simulink model "main"  (R2016b)
settings: Solver=VariableStepAuto  StartTime=0.0  StopTime=40  FixedStep=Par.Step_size  RelTol=1e-3
values from neighbouring files (symbols this model uses):
  eta_0 = [0 0 0]    [K_psi_test.m]
  nu_0 = [0 0 0]    [K_psi_test.m]
undefined symbols (not defined in the file or in its folder): now, Par
libraries: simulink x4
settings Model: Creator=Ørjan  LastModifiedBy=Ørjan
settings DataIOCC: SaveState=on  ReturnWorkspaceOutputs=on  ReturnWorkspaceOutputsName=spidata
settings RTWCC: RTWCompilerOptimization=on
settings CodeAppCC: MaxIdLength=95

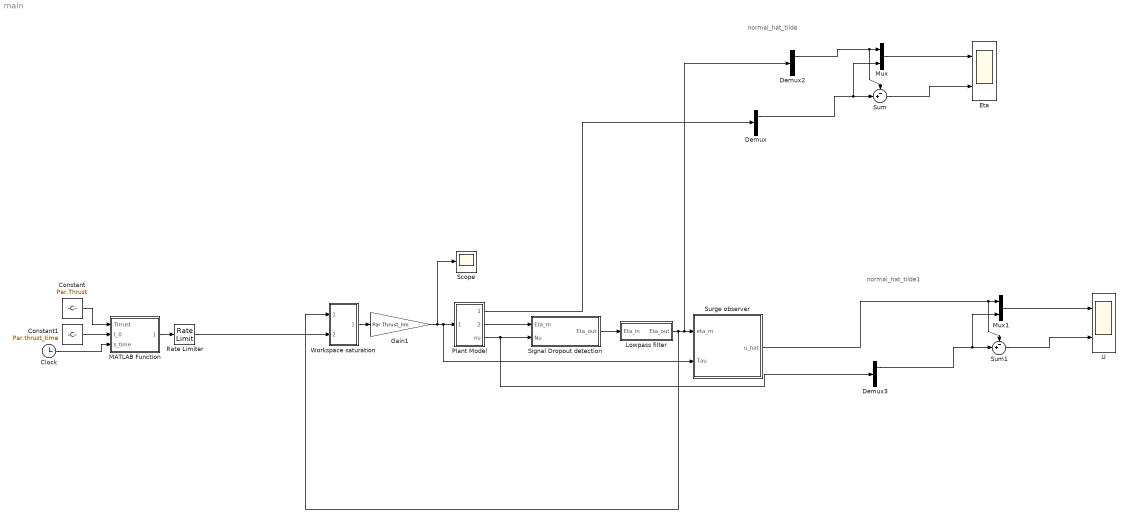
== system main ==
  note: normal_hat_tilde1
  note: normal_hat_tilde
  Clock : Clock
  Constant : Constant  Value=Par.Thrust  VectorParams1D=off
  Constant1 : Constant  Value=Par.thrust_time
  Demux : Demux  Outputs=3
  Demux2 : Demux  Outputs=3
  Demux3 : Demux  Outputs=3
  Eta : Scope  NumInputPorts=2
  Gain1 : Gain  Gain=Par.Thrust_lim
  Lowpass filter : Subsystem
  MATLAB Function : MATLAB Function  TreatAsAtomicUnit=on
  Mux : Mux  Inputs=2
  Mux1 : Mux  Inputs=2
  Plant Model : Subsystem
  Rate Limiter : RateLimiter  RisingSlewLimit=5  FallingSlewLimit=-5  SampleTimeMode=inherited
  Scope : Scope
  Signal Dropout detection : Subsystem
  Sum : Sum  Inputs=-+|
  Sum1 : Sum  Inputs=-+|
  Surge observer : Subsystem
  U : Scope  NumInputPorts=2
  Workspace saturation : Subsystem
  wires:
  Constant/1 -> MATLAB Function/1(Thrust)
  Clock/1 -> MATLAB Function/3(s_time)
  MATLAB Function/1(tau_norm) -> Rate Limiter/1
  Rate Limiter/1 -> Workspace saturation/2(Tau_in)
  Workspace saturation/1(Tau_out) -> Gain1/1
  Plant Model/2(eta_m) -> Signal Dropout detection/1(Eta_m)
  Signal Dropout detection/1(Eta_out) -> Lowpass filter/1(Eta_in)
  Gain1/1 -> Scope/1, Surge observer/2(Tau), Plant Model/1(tau)
  Lowpass filter/1(Eta_out) -> Workspace saturation/1(Eta_in), Demux2/1, Surge observer/1(eta_m)
  Plant Model/1(eta) -> Demux/1
  Demux/1 -> Mux/2, Sum/2
  Sum/1 -> Eta/2
  Demux2/1 -> Sum/1, Mux/1
  Mux/1 -> Eta/1
  Plant Model/3(nu) -> Demux3/1, Signal Dropout detection/2(Nu)
  Demux3/1 -> Mux1/2, Sum1/2
  Sum1/1 -> U/2
  Surge observer/1(u_hat) -> Sum1/1, Mux1/1
  Mux1/1 -> U/1
  Constant1/1 -> MATLAB Function/2(t_0)

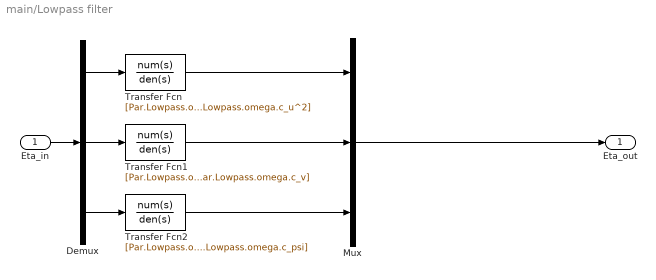
== system main/Lowpass filter ==
  Eta_in : Inport
  Demux : Demux  Outputs=3
  Mux : Mux  Inputs=3
  Transfer Fcn : TransferFcn  Numerator=[Par.Lowpass.omega.c_u^2]  Denominator=[1 Par.Lowpass.omega.c_u Par.Lowpass.omega.c_u^2]
  Transfer Fcn1 : TransferFcn  Numerator=[Par.Lowpass.omega.c_v]  Denominator=[1 Par.Lowpass.omega.c_v]
  Transfer Fcn2 : TransferFcn  Numerator=[Par.Lowpass.omega.c_psi]  Denominator=[1 Par.Lowpass.omega.c_psi]
  Eta_out : Outport
  wires:
  Eta_in/1 -> Demux/1
  Demux/1 -> Transfer Fcn/1
  Demux/2 -> Transfer Fcn1/1
  Demux/3 -> Transfer Fcn2/1
  Transfer Fcn2/1 -> Mux/3
  Transfer Fcn1/1 -> Mux/2
  Transfer Fcn/1 -> Mux/1
  Mux/1 -> Eta_out/1

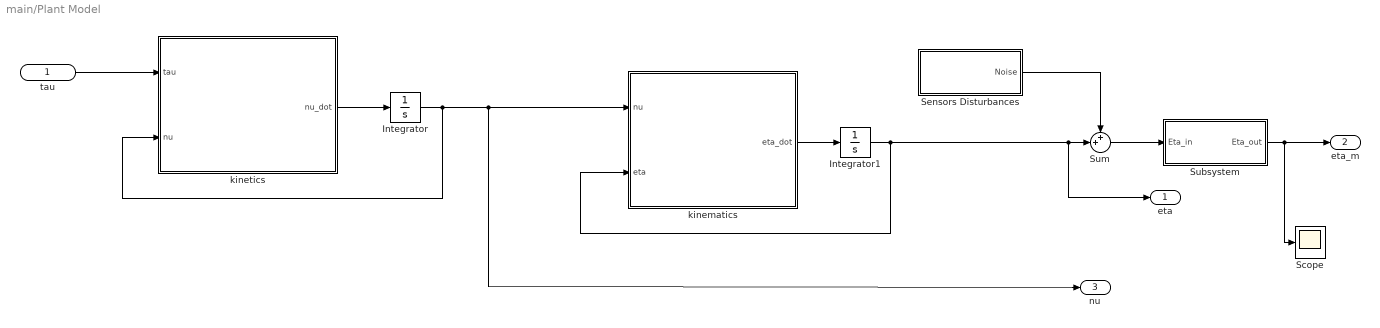
== system main/Plant Model ==
  tau : Inport
  Integrator : Integrator  InitialCondition=nu_0
  Integrator1 : Integrator  InitialCondition=eta_0
  Scope : Scope
  Sensors Disturbances : Subsystem
  Subsystem : Subsystem
  Sum : Sum  Inputs=++|
  kinematics : MATLAB Function  TreatAsAtomicUnit=on
  kinetics : MATLAB Function  TreatAsAtomicUnit=on
  eta : Outport
  eta_m : Outport  Port=2
  nu : Outport  Port=3
  wires:
  tau/1 -> kinetics/1(tau)
  kinetics/1(nu_dot) -> Integrator/1
  kinematics/1(eta_dot) -> Integrator1/1
  Integrator/1 -> kinetics/2(nu), nu/1, kinematics/1(nu)
  Integrator1/1 -> eta/1, Sum/2, kinematics/2(eta)
  Sensors Disturbances/1(Noise) -> Sum/1
  Subsystem/1(Eta_out) -> Scope/1, eta_m/1
  Sum/1 -> Subsystem/1(Eta_in)

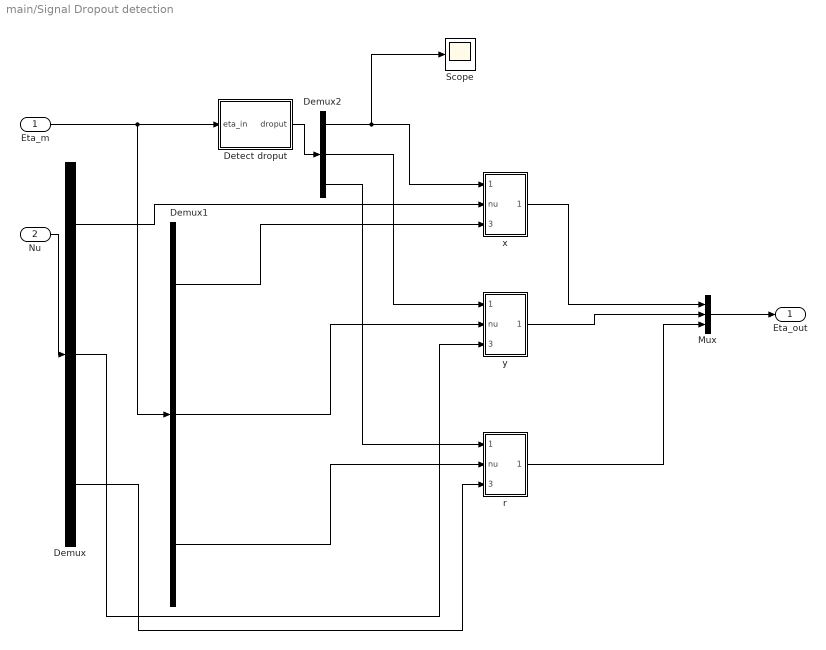
== system main/Signal Dropout detection ==
  Eta_m : Inport
  Nu : Inport  Port=2
  Demux : Demux  Outputs=3
  Demux1 : Demux  Outputs=3
  Demux2 : Demux  Outputs=3
  Detect droput : MATLAB Function  TreatAsAtomicUnit=on
  Mux : Mux  Inputs=3
  Scope : Scope
  r : Subsystem
  x : Subsystem
  y : Subsystem
  Eta_out : Outport
  wires:
  Nu/1 -> Demux/1
  Eta_m/1 -> Detect droput/1(eta_in), Demux1/1
  Detect droput/1(droput) -> Demux2/1
  y/1(new_eta) -> Mux/2
  r/1(new_eta) -> Mux/3
  Mux/1 -> Eta_out/1
  Demux2/1 -> Scope/1, x/1(detect droput)
  Demux/1 -> x/2(nu)
  Demux1/1 -> x/3(eta)
  x/1(new_eta) -> Mux/1
  Demux1/2 -> y/2(nu)
  Demux2/2 -> y/1(detect droput)
  Demux2/3 -> r/1(detect droput)
  Demux1/3 -> r/2(nu)
  Demux/2 -> y/3(eta)
  Demux/3 -> r/3(eta)

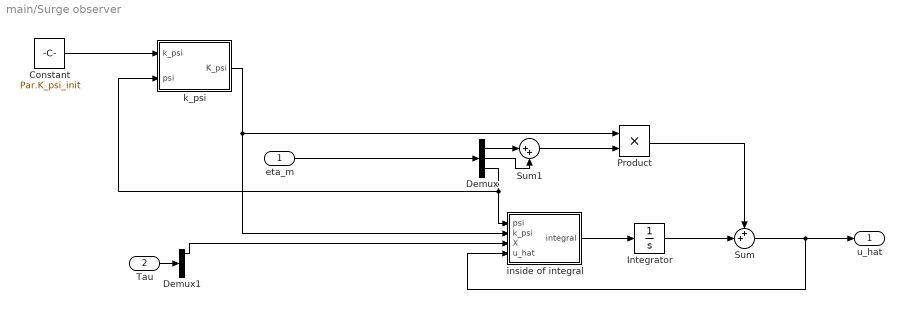
== system main/Surge observer ==
  eta_m : Inport
  Tau : Inport  Port=2
  Constant : Constant  Value=Par.K_psi_init
  Demux : Demux  Outputs=3
  Demux1 : Demux  Outputs=3
  Integrator : Integrator
  Product : Product
  Sum : Sum  Inputs=++|
  Sum1 : Sum  Inputs=|++
  inside of integral : MATLAB Function  TreatAsAtomicUnit=on
  k_psi : MATLAB Function  TreatAsAtomicUnit=on
  u_hat : Outport
  wires:
  inside of integral/1(integral) -> Integrator/1
  k_psi/1(K_psi) -> Product/1, inside of integral/2(k_psi)
  Integrator/1 -> Sum/2
  Tau/1 -> Demux1/1
  Demux1/1 -> inside of integral/3(X)
  Demux/3 -> k_psi/2(psi), inside of integral/1(psi)
  Sum/1 -> inside of integral/4(u_hat), u_hat/1
  Demux/1 -> Sum1/1
  Demux/2 -> Sum1/2
  Sum1/1 -> Product/2
  Product/1 -> Sum/1
  eta_m/1 -> Demux/1
  Constant/1 -> k_psi/1(k_psi)

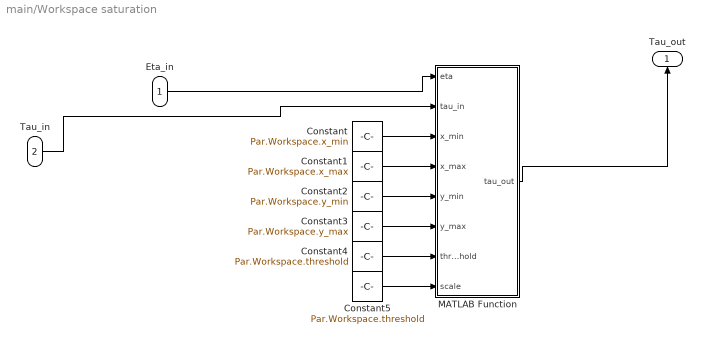
== system main/Workspace saturation ==
  Eta_in : Inport
  Tau_in : Inport  Port=2
  Constant : Constant  Value=Par.Workspace.x_min
  Constant1 : Constant  Value=Par.Workspace.x_max
  Constant2 : Constant  Value=Par.Workspace.y_min
  Constant3 : Constant  Value=Par.Workspace.y_max
  Constant4 : Constant  Value=Par.Workspace.threshold
  Constant5 : Constant  Value=Par.Workspace.threshold
  MATLAB Function : MATLAB Function  TreatAsAtomicUnit=on
  Tau_out : Outport
  wires:
  Constant3/1 -> MATLAB Function/6(y_max)
  Constant/1 -> MATLAB Function/3(x_min)
  Constant4/1 -> MATLAB Function/7(threshold)
  Constant2/1 -> MATLAB Function/5(y_min)
  Constant1/1 -> MATLAB Function/4(x_max)
  Eta_in/1 -> MATLAB Function/1(eta)
  Tau_in/1 -> MATLAB Function/2(tau_in)
  MATLAB Function/1(tau_out) -> Tau_out/1
  Constant5/1 -> MATLAB Function/8(scale)

== system main/Plant Model/Sensors Disturbances ==
  Band-Limited White Noise : simulink/Sources/Band-Limited White Noise  Cov=Par.Noise.Power  Ts=Par.Noise.Sample_time  seed=ceil(abs(3*round(abs(now*1e6 - fix(now*1e6))*1e5)))
  Constant : Constant  Value=[0 0 0]
  Par.SensNoiseEnabled : Constant  Value=Par.SensNoiseEnabled
  Switch : Switch  Criteria=u2 > Threshold
  Noise : Outport
  wires:
  Par.SensNoiseEnabled/1 -> Switch/2
  Switch/1 -> Noise/1
  Constant/1 -> Switch/3
  Band-Limited White Noise/1 -> Switch/1

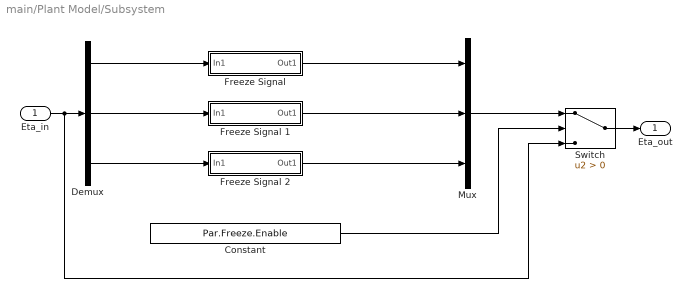
== system main/Plant Model/Subsystem ==
  Eta_in : Inport
  Constant : Constant  Value=Par.Freeze.Enable
  Demux : Demux  Outputs=3
  "Freeze Signal " : Subsystem
  Freeze Signal 1 : Subsystem
  Freeze Signal 2 : Subsystem
  Mux : Mux  Inputs=3
  Switch : Switch  Criteria=u2 > Threshold
  Eta_out : Outport
  wires:
  Eta_in/1 -> Switch/3, Demux/1
  Mux/1 -> Switch/1
  Demux/1 -> "Freeze Signal "/1(In1)
  "Freeze Signal "/1(Out1) -> Mux/1
  Freeze Signal 1/1(Out1) -> Mux/2
  Demux/2 -> Freeze Signal 1/1(In1)
  Demux/3 -> Freeze Signal 2/1(In1)
  Freeze Signal 2/1(Out1) -> Mux/3
  Constant/1 -> Switch/2
  Switch/1 -> Eta_out/1

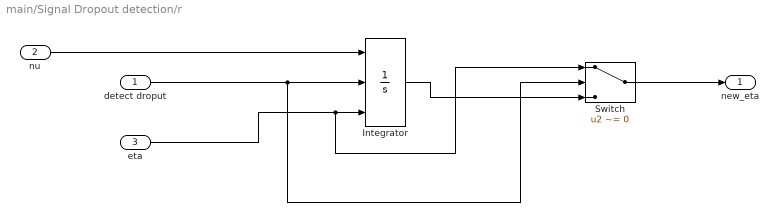
== system main/Signal Dropout detection/r ==
  detect droput : Inport
  nu : Inport  Port=2
  eta : Inport  Port=3
  Integrator : Integrator  ExternalReset=rising  InitialConditionSource=external
  Switch : Switch  Criteria=u2 ~= 0
  new_eta : Outport
  wires:
  Switch/1 -> new_eta/1
  nu/1 -> Integrator/1
  eta/1 -> Switch/1, Integrator/3
  detect droput/1 -> Switch/2, Integrator/2
  Integrator/1 -> Switch/3

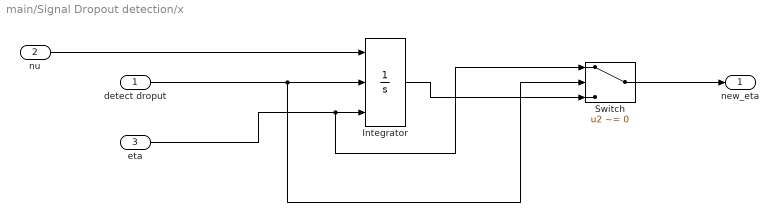
== system main/Signal Dropout detection/x ==
  detect droput : Inport
  nu : Inport  Port=2
  eta : Inport  Port=3
  Integrator : Integrator  ExternalReset=rising  InitialConditionSource=external
  Switch : Switch  Criteria=u2 ~= 0
  new_eta : Outport
  wires:
  Switch/1 -> new_eta/1
  nu/1 -> Integrator/1
  eta/1 -> Switch/1, Integrator/3
  detect droput/1 -> Switch/2, Integrator/2
  Integrator/1 -> Switch/3

== system main/Signal Dropout detection/y ==
  detect droput : Inport
  nu : Inport  Port=2
  eta : Inport  Port=3
  Integrator : Integrator  ExternalReset=rising  InitialConditionSource=external
  Switch : Switch  Criteria=u2 ~= 0
  new_eta : Outport
  wires:
  Switch/1 -> new_eta/1
  nu/1 -> Integrator/1
  eta/1 -> Switch/1, Integrator/3
  detect droput/1 -> Switch/2, Integrator/2
  Integrator/1 -> Switch/3

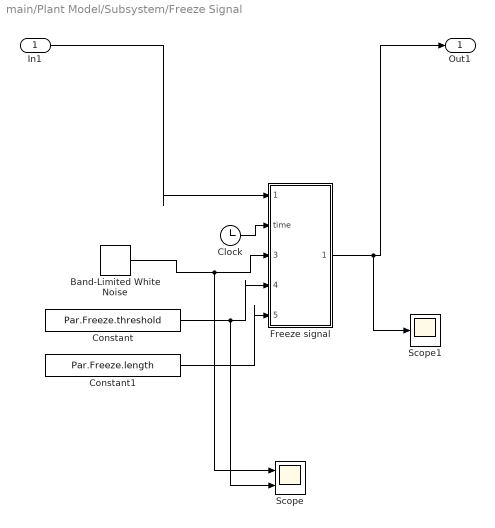
== system main/Plant Model/Subsystem/Freeze Signal  ==
  In1 : Inport
  Band-Limited White Noise : simulink/Sources/Band-Limited White Noise  Cov=Par.Freeze.Power  Ts=Par.Noise.Sample_time  seed=ceil(abs(5*round(abs(now*1e6 - fix(now*1e6))*1e5)))
  Clock : Clock
  Constant : Constant  Value=Par.Freeze.threshold
  Constant1 : Constant  Value=Par.Freeze.length
  Freeze signal : MATLAB Function  TreatAsAtomicUnit=on
  Scope : Scope  NumInputPorts=2
  Scope1 : Scope
  Out1 : Outport
  wires:
  Constant1/1 -> Freeze signal/5(length)
  In1/1 -> Freeze signal/1(eta_in)
  Freeze signal/1(eta_out) -> Scope1/1, Out1/1
  Constant/1 -> Scope/2, Freeze signal/4(threshold)
  Clock/1 -> Freeze signal/2(time)
  Band-Limited White Noise/1 -> Scope/1, Freeze signal/3(random_value)

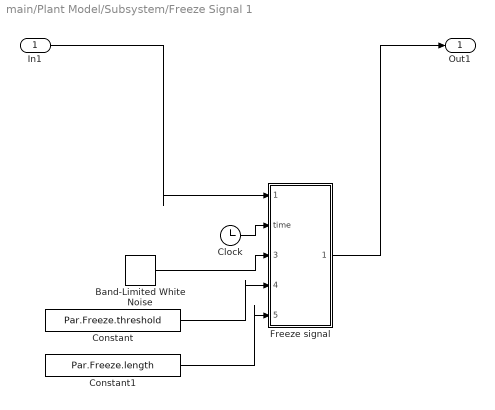
== system main/Plant Model/Subsystem/Freeze Signal 1 ==
  In1 : Inport
  Band-Limited White Noise : simulink/Sources/Band-Limited White Noise  Cov=Par.Freeze.Power  Ts=Par.Noise.Sample_time  seed=ceil(abs(5*round(abs(now*1e6 - fix(now*1e6))*1e5)))
  Clock : Clock
  Constant : Constant  Value=Par.Freeze.threshold
  Constant1 : Constant  Value=Par.Freeze.length
  Freeze signal : MATLAB Function  TreatAsAtomicUnit=on
  Out1 : Outport
  wires:
  Constant1/1 -> Freeze signal/5(length)
  In1/1 -> Freeze signal/1(eta_in)
  Freeze signal/1(eta_out) -> Out1/1
  Constant/1 -> Freeze signal/4(threshold)
  Clock/1 -> Freeze signal/2(time)
  Band-Limited White Noise/1 -> Freeze signal/3(random_value)

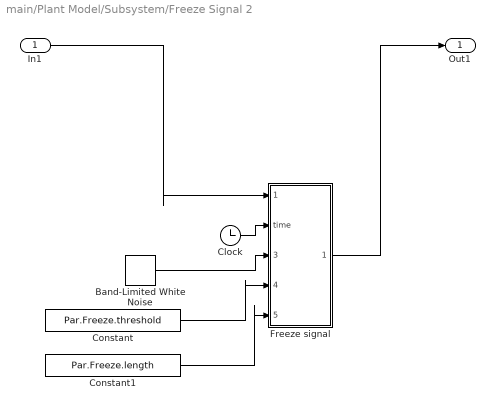
== system main/Plant Model/Subsystem/Freeze Signal 2 ==
  In1 : Inport
  Band-Limited White Noise : simulink/Sources/Band-Limited White Noise  Cov=Par.Freeze.Power  Ts=Par.Noise.Sample_time  seed=ceil(abs(5*round(abs(now*1e6 - fix(now*1e6))*1e5)))
  Clock : Clock
  Constant : Constant  Value=Par.Freeze.threshold
  Constant1 : Constant  Value=Par.Freeze.length
  Freeze signal : MATLAB Function  TreatAsAtomicUnit=on
  Out1 : Outport
  wires:
  Constant1/1 -> Freeze signal/5(length)
  In1/1 -> Freeze signal/1(eta_in)
  Freeze signal/1(eta_out) -> Out1/1
  Constant/1 -> Freeze signal/4(threshold)
  Clock/1 -> Freeze signal/2(time)
  Band-Limited White Noise/1 -> Freeze signal/3(random_value)

== matlab function main/Plant Model/kinematics ==
  data: nu input; eta_dot output; eta input
function eta_dot = CSE1_eta_dot(nu,eta)

psi = eta(3);

J = [cos(psi) -sin(psi) 0
     sin(psi) cos(psi)  0
     0        0         1];

eta_dot = J*nu;

== matlab function main/Plant Model/kinetics ==
  data: tau input; nu_dot output; nu input
function nu_dot = CSE1_nu_dot(tau,nu)

u   = nu(1);
v   = nu(2);
r   = nu(3);

tau = [tau(1);tau(2);tau(3)];
%% MATRICES

m    = 14.79;   I_z  =  1.7600;   x_g = 0.0375;       % x_g  =  0.0460; % Table B.1


%% Added mass
X_ud  =     -2.0;											% Table B.1
					Y_vd =     -1.0;	N_vd =    -0.0;		% Table B.1 guestimate
					Y_rd =      -0.0;	N_rd =    -1.0;		% Table B.1

%% Total mass matrix
m_11 = m-X_ud;
m_22 = m-Y_vd;
m_23 = m*x_g-Y_rd;
m_32 = m*x_g-N_vd;
m_33 = I_z-N_rd;

M    = [m_11 0    0
        0    m_22 m_23
        0    m_32 m_33];
	
%% Damping coefficients
% Comments at the end of the lines indicate the old values used.
X_u		= -0.6555;		X_v		= 0;
X_uu 	= 0.3545;		X_vv	= -2.443;
X_uuu 	= -3.787;		X_vvv	= 0;

						Y_v		= -1.33; 			Y_r		= -7.250; % Y_r
						Y_vv	= -2.776;			Y_rr	= -3.450; % Y_rr
						Y_vvv	= -64.91;			Y_rrr	= 0;
						
						Y_rv	= -0.805;			Y_vr	= -0.845; % Y_rv, Y_vr

						N_v		= 0;				N_r		= -1.900; % N_r
						N_vv	= -0.2088;			N_rr	= -0.750; % N_rr
						N_vvv	= 0;				N_rrr	= 0;
						
						N_rv	= 0.130;			N_vr	= 0.080; % N_rv, N_vr

%% Correolis matrix
c_13 = -(m-Y_vd)*v-(m*x_g-Y_rd)*r;
c_23 = (m-X_ud)*u;
C    = [0     0     c_13
        0     0     c_23
        -c_13 -c_23 0   ];

%% Assembly of the damping matrix
d_11 = -X_u - X_uu*u - X_uuu*u^2;
d_22 = -Y_v - Y_vv*v - Y_vvv*v^2 - Y_rv*abs(r);
d_33 = -N_r - N_rr*abs(r) - N_rrr*r^2 - N_vr*abs(v); % using abs(r)

d_12 = -X_v - X_vv*v - X_vvv*v^2;
d_23 = -Y_r - Y_rr*abs(r) - Y_rrr*r^2 - Y_vr*abs(v);
d_32 = -N_v - N_vv*v - N_vvv*v^2 - N_rv*abs(r);

D    = [d_11 d_12 0
        0    d_22 d_23
        0    d_32 d_33];



%% CALCULATION
nu_dot = M\(tau-(C+D)*nu);

== matlab function main/Workspace saturation/MATLAB Function ==
  data: eta input; tau_out output; tau_in input; x_min input; x_max input; y_min input; y_max input; threshold input; scale input
function tau_out = fcn(eta, tau_in, x_min, x_max, y_min, y_max, threshold, scale)
%#codegen
R = [cos(eta(3)) sin(eta(3)) 0 ; -sin(eta(3)) cos(eta(3)) 0; 0 0 1];

tau_NED = R*tau_in;
tau_NED_out = tau_NED;

%check if x is above limits
if (eta(1) > x_max)
    %x is above of the limit
    epsilon = ((eta(1) - x_max)/threshold);
    tau_NED_out(1) = -epsilon;% + tau_NED(1)*(1-epsilon);
end
%check if x is below limits
if (eta(1) < x_min)
    %x is below of the limit
    epsilon = ((eta(1) - x_min)/threshold);
    tau_NED_out(1) = -epsilon;% + tau_NED(1)*(1+epsilon);
end
%check if y is above limits
if (eta(2) > y_max)
    %x is above of the limit
    epsilon = ((eta(2) - y_max)/threshold);
    tau_NED_out(2) = -epsilon;% + tau_NED(2)*(1-epsilon);
end
%check if y is above limits
if (eta(2) < y_min)
    %x is above of the limit
    epsilon = ((eta(2) - y_min)/threshold);
    tau_NED_out(2) = -epsilon;% + tau_NED(2)*(1+epsilon);
end
tau_out = R'*tau_NED_out;
end

== matlab function main/MATLAB Function ==
  data: tau_norm output; Thrust input; t_0 input; s_time input
function tau_norm = fcn(Thrust, t_0, s_time)
%coder.extrinsic('get_param');
tau_norm = zeros(3,1);
persistent i;
persistent tau;
if(isempty(i))
    i = 1;
end
if(isempty(tau))
    tau = [0; 0; 0];
end
if(s_time>t_0(i))
    tau(1) = Thrust(i, 1);
    tau(2) = Thrust(i, 2);
    tau(3) = Thrust(i, 3);
    if(i<size(Thrust, 1))
        i = i +1;
    end
end
tau_norm = tau;
end

== matlab function main/Surge observer/inside of integral ==
  data: psi input; k_psi input; X input; u_hat input; integral output
function integral = fcn(psi, k_psi, X, u_hat)
%#codegen
X_u = -.6555;
X_uu = .3545;
X_uuu = -3.787;
m_11 = 16.79;
d_11 = -X_u -X_uu*abs(u_hat) - X_uuu*u_hat^2;
integral = -d_11*u_hat/m_11 + X/m_11 - k_psi*(cos(psi) + sin(psi))*u_hat;
end

== matlab function main/Surge observer/k_psi ==
  data: k_psi input; psi input; K_psi output
function K_psi = fcn(k_psi, psi)
%#codegen
K_psi = k_psi*sign(sin(psi) + cos(psi));
% y = u;

== matlab function main/Signal Dropout detection/Detect droput ==
  data: eta_in input; droput output
function droput = fcn(eta_in)
persistent eta_old;
persistent i;
if isempty(eta_old)
    eta_old = zeros(3, 5);
end
if isempty(i)
    i = 1;
end
eta_old(1:3, i) = eta_in;
i = i+1;
if(i==6)
    i = 1;
end

droput = (eta_in - sum(eta_old')'/5) == 0;

end

== matlab function main/Plant Model/Subsystem/Freeze Signal /Freeze signal ==
  data: eta_in input; eta_out output; time input; random_value input; threshold input; length input
function eta_out = fcn(eta_in, time, random_value, threshold, length)
persistent eta t_1;
if isempty(eta)
    eta = eta_in;
    t_1 = 0;
end

if random_value > threshold
    t_1 = time + length*(0.5*rand+0.5);
end
if time>=t_1
    eta = eta_in;
end

eta_out = eta;
end

== matlab function main/Plant Model/Subsystem/Freeze Signal 1/Freeze signal ==
  data: eta_in input; eta_out output; time input; random_value input; threshold input; length input
function eta_out = fcn(eta_in, time, random_value, threshold, length)
persistent eta t_1;
if isempty(eta)
    eta = eta_in;
    t_1 = 0;
end

if random_value > threshold
    t_1 = time + length*(0.5*rand+0.5);
end
if time>=t_1
    eta = eta_in;
end

eta_out = eta;
end

== matlab function main/Plant Model/Subsystem/Freeze Signal 2/Freeze signal ==
  data: eta_in input; eta_out output; time input; random_value input; threshold input; length input
function eta_out = fcn(eta_in, time, random_value, threshold, length)
persistent eta t_1;
if isempty(eta)
    eta = eta_in;
    t_1 = 0;
end

if random_value > threshold
    t_1 = time + length*(0.5*rand+0.5);
end
if time>=t_1
    eta = eta_in;
end

eta_out = eta;
end
